simulink model "code_group46"  (R2022b)
settings: Solver=FixedStepAuto  StartTime=0.0  StopTime=2  FixedStep=1e-3  RelTol=1e-3  EnableMultiTasking=on
undefined symbols (not defined in the file): A0, A1, D0, D1, D10, D11, D12, D13, D2, D3, D4, D5, D6, D7, D8, D9, PTA0, PTA1, PTA2, PTB2, PTB23, PTB3, PTB9, PTC16, PTC17, PTC2, PTC3, PTC4, PTD0, PTD1, PTD2, PTD3
libraries: frdmk64flib x19, etargetslib x19, simulink x2
(part 1 of 2)
settings Model: ExtModeTrigDuration=5  Creator=aliciamorielli  LastModifiedBy=kavya
settings SolverCC: AlgebraicLoopSolver=TrustRegion
settings OptimizationCC: EnhancedBackFolding=on  PassReuseOutputArgsThreshold=0  MaxStackSize=64  OptimizeBlockOrder=speed  DifferentSizesBufferReuse=on  OptimizationCustomize=off
settings DebuggingCC: ParameterTunabilityLossMsg=error  UnconnectedInputMsg=warning  UnconnectedOutputMsg=warning  UnconnectedLineMsg=warning  SFMachineParentedDataDiag=warning
settings HardwareCC: ProdBitPerPointer=32  ProdBitPerSizeT=32  ProdBitPerPtrDiffT=32  ProdLargestAtomicInteger=Long  ProdLargestAtomicFloat=Double  ProdWordSize=32  ProdHWDeviceType=ARM Compatible->ARM Cortex  UseEmbeddedCoderFeatures=off
settings ModelReferenceCC: EnableRefExpFcnMdlSchedulingChecks=on
settings SFSimCC: MATLABDynamicMemAlloc=off
settings RTWCC: Description=Embedded Coder  SystemTargetFile=ert.tlc  HardwareBoard=NXP FRDM-K64F  TLCOptions="-aInlineSetEventsForThisBaseRateFcn=TLC_FALSE -aSuppressMultiTaskScheduler=TLC_FALSE  -aRateBasedStepFcn=0"  TemplateMakefile=ert_default_tmf  Toolchain=GNU Tools for ARM Embedded Processors  DLArmComputeVersion=19.05
settings CodeAppCC: ForceParamTrailComments=on  OperatorAnnotations=on
settings ERTTargetCC: ERTCustomFileBanners=off  SupportContinuousTime=on  SupportNonInlinedSFcns=on  RemoveResetFunc=off  ModelStepFunctionPrototypeControlCompliant=off  ExtModeTransport=4  ExtModeMexFile=sendToCommService

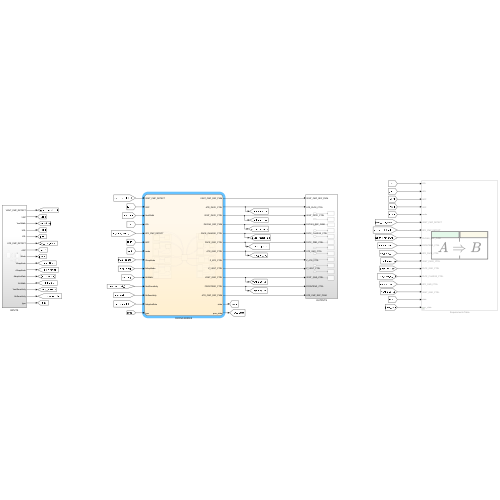
[thumbnail: Simulink's stored preview of the top-level diagram]
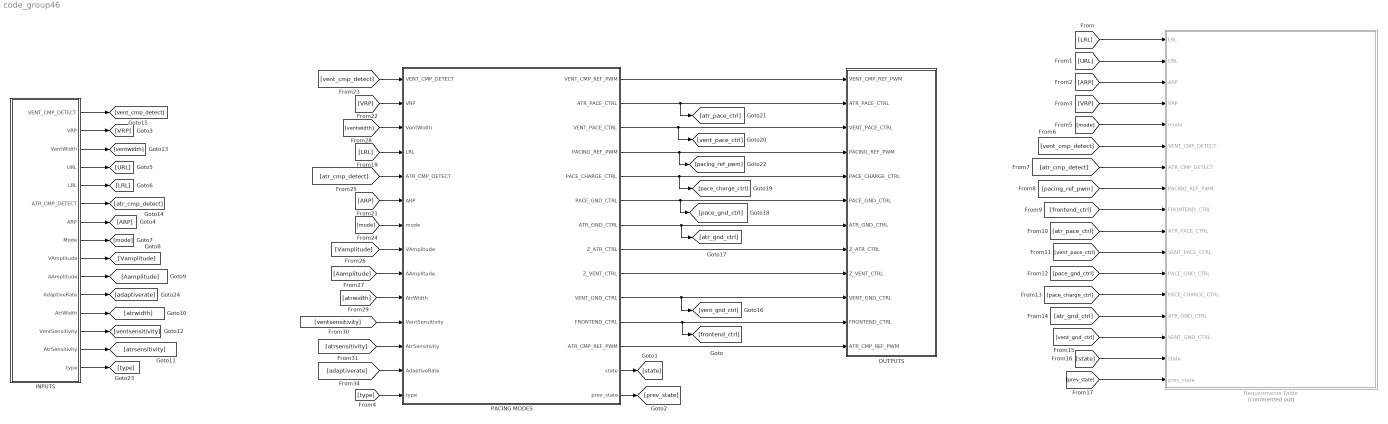
== system code_group46 ==
  INPUTS : Subsystem
  OUTPUTS : Subsystem
  PACING MODES : Stateflow chart  TreatAsAtomicUnit=on
      settings: PortSchema="{\"entries\":[{\"content\":{\"sides\":[{\"content\":{\"connectorIds\":[\"In1\",\"In4\",\"In2\",\"In3\",\"In6\",\"In5\",\"In7\",\"In8\",\"In9\",\"In10\",\"In11\",\"In12\",\"In13\",\"In14\"]},\"type\":\"ConnectorPlacement.EquallySpacedRectSide\",\"uuid\":\"24afec03-bc13-4065-9064-27bef3c43f7a\"},{\"content\":{\"connectorIds\":[\"Out11\",\"Out1\",\"Out2\",\"Out3\",\"Out4\",\"Out5\",\"Out6\",\"Out7\",\"Out8\",\"Out9\",\"Out10\",\"Out12\",\"Out13\",\"Out14\"],\"side\":\"RIGHT\"},\"type\":\"ConnectorPlacement.EquallySpacedRectSide\",\"uuid\":\"79d0ee85-df22-4c09-8ba8-cd763efde854\"},{\"content\":{\"connectorIds\":[],\"side\":\"TOP\"},\"type\":\"ConnectorPlacement.EquallySpacedRectSide\",\"uuid\":\"d342e713-b0ae-4b06-a4c2-9648f7d82d61\"},{\"content\":{\"connectorIds\":[],\"side\":\"BOTTOM\"},\"type\":\"ConnectorPlacement.EquallySpacedRectSide\",\"uuid\":\"4b63818c-7bd6-427f-a568-d3913931a17b\"}]},\"type\":\"ConnectorPlacement.EquallySpacedConnector\",\"uuid\":\"408ec0d3-1c59-4342-b3c9-42fd185f3962\"}],\"packageUris\":[\"http://schema.mathworks.com/mf0/Connector/R2020b\"],\"version\":\"1.0\"}"
  Requirements Table : Requirements Table  Commented=on  TreatAsAtomicUnit=on
  wires:
  PACING MODES/11(VENT_CMP_REF_PWM) -> OUTPUTS/1(VENT_CMP_REF_PWM)
  PACING MODES/2(VENT_PACE_CTRL) -> [vent_pace_ctrl], OUTPUTS/3(VENT_PACE_CTRL)
  PACING MODES/3(PACING_REF_PWM) -> [pacing_ref_pwm], OUTPUTS/4(PACING_REF_PWM)
  PACING MODES/4(PACE_CHARGE_CTRL) -> [pace_charge_ctrl], OUTPUTS/5(PACE_CHARGE_CTRL)
  PACING MODES/5(PACE_GND_CTRL) -> [pace_gnd_ctrl], OUTPUTS/6(PACE_GND_CTRL)
  PACING MODES/6(ATR_GND_CTRL) -> [atr_gnd_ctrl], OUTPUTS/7(ATR_GND_CTRL)
  PACING MODES/7(Z_ATR_CTRL) -> OUTPUTS/8(Z_ATR_CTRL)
  PACING MODES/8(Z_VENT_CTRL) -> OUTPUTS/9(Z_VENT_CTRL)
  PACING MODES/9(VENT_GND_CTRL) -> [vent_gnd_ctrl], OUTPUTS/10(VENT_GND_CTRL)
  PACING MODES/10(FRONTEND_CTRL) -> [frontend_ctrl], OUTPUTS/11(FRONTEND_CTRL)
  PACING MODES/12(ATR_CMP_REF_PWM) -> OUTPUTS/12(ATR_CMP_REF_PWM)
  PACING MODES/1(ATR_PACE_CTRL) -> [atr_pace_ctrl], OUTPUTS/2(ATR_PACE_CTRL)
  [LRL] -> Requirements Table/1(LRL)
  [URL] -> Requirements Table/2(URL)
  [ARP] -> Requirements Table/3(ARP)
  [VRP] -> Requirements Table/4(VRP)
  [mode] -> Requirements Table/5(mode)
  [vent_cmp_detect] -> Requirements Table/6(VENT_CMP_DETECT)
  [atr_cmp_detect] -> Requirements Table/7(ATR_CMP_DETECT)
  [pacing_ref_pwm] -> Requirements Table/8(PACING_REF_PWM)
  [frontend_ctrl] -> Requirements Table/9(FRONTEND_CTRL)
  [atr_pace_ctrl] -> Requirements Table/10(ATR_PACE_CTRL)
  [vent_pace_ctrl] -> Requirements Table/11(VENT_PACE_CTRL)
  [pace_gnd_ctrl] -> Requirements Table/12(PACE_GND_CTRL)
  [pace_charge_ctrl] -> Requirements Table/13(PACE_CHARGE_CTRL)
  [atr_gnd_ctrl] -> Requirements Table/14(ATR_GND_CTRL)
  [vent_gnd_ctrl] -> Requirements Table/15(VENT_GND_CTRL)
  [state] -> Requirements Table/16(state)
  [prev_state] -> Requirements Table/17(prev_state)
  PACING MODES/13(state) -> [state]
  PACING MODES/14(prev_state) -> [prev_state]
  [LRL] -> PACING MODES/3(LRL)
  [ARP] -> PACING MODES/5(ARP)
  [VRP] -> PACING MODES/4(VRP)
  [mode] -> PACING MODES/7(mode)
  [vent_cmp_detect] -> PACING MODES/1(VENT_CMP_DETECT)
  [atr_cmp_detect] -> PACING MODES/6(ATR_CMP_DETECT)
  [Vamplitude] -> PACING MODES/8(VAmplitude)
  [Aamplitude] -> PACING MODES/9(AAmplitude)
  INPUTS/2(VRP) -> [VRP]
  INPUTS/7(ARP) -> [ARP]
  INPUTS/3(VentWidth) -> [ventwidth]
  INPUTS/5(LRL) -> [LRL]
  INPUTS/8(Mode) -> [mode]
  INPUTS/9(VAmplitude) -> [Vamplitude]
  INPUTS/10(AAmplitude) -> [Aamplitude]
  INPUTS/13(VentSensitivity) -> [ventsensitivity]
  INPUTS/14(AtrSensitivity) -> [atrsensitivity]
  INPUTS/12(AtrWidth) -> [atrwidth]
  [ventwidth] -> PACING MODES/2(VentWidth)
  [atrwidth] -> PACING MODES/10(AtrWidth)
  INPUTS/1(VENT_CMP_DETECT) -> [vent_cmp_detect]
  INPUTS/6(ATR_CMP_DETECT) -> [atr_cmp_detect]
  [ventsensitivity] -> PACING MODES/11(VentSensitivity)
  [atrsensitivity] -> PACING MODES/12(AtrSensitivity)
  INPUTS/4(URL) -> [URL]
  INPUTS/11(AdaptiveRate) -> [adaptiverate]
  [adaptiverate] -> PACING MODES/13(AdaptiveRate)
  [type] -> PACING MODES/14(type)
  INPUTS/15(type) -> [type]

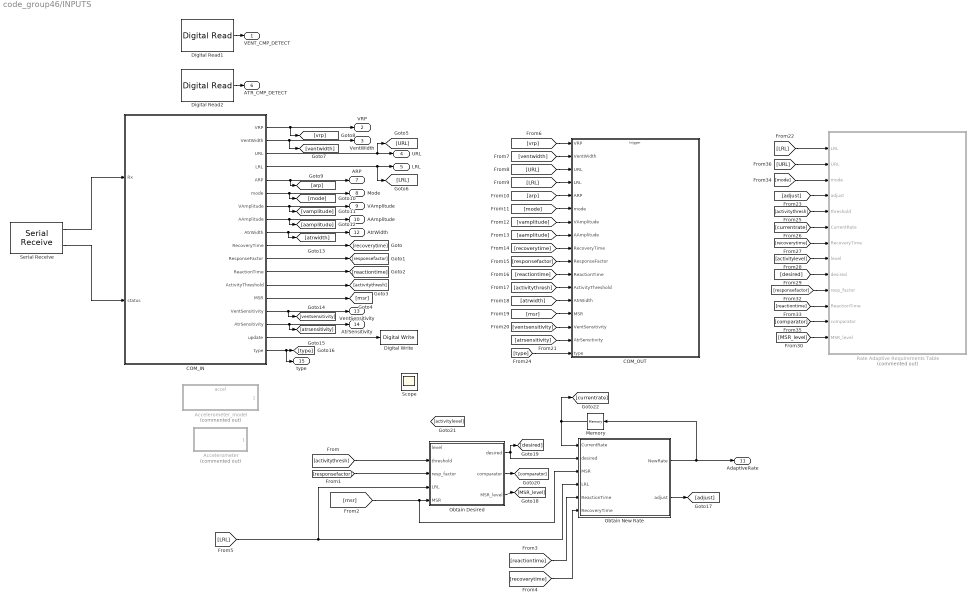
== system code_group46/INPUTS ==
  Accelerometer : Subsystem  Commented=on  ReferencedSubsystem=accelerometer
  Accelerometer_model : ModelReference  Commented=on  ModelNameDialog=accel  SimulationMode=Normal  ModelReferenceVersion=2.0
  COM_IN : Stateflow chart  TreatAsAtomicUnit=on
      settings: PortSchema="{\"entries\":[{\"content\":{\"sides\":[{\"content\":{\"connectorIds\":[\"In1\",\"In2\"]},\"type\":\"ConnectorPlacement.EquallySpacedRectSide\",\"uuid\":\"eafe7878-2647-49a4-97cb-41e68478fa40\"},{\"content\":{\"connectorIds\":[\"Out3\",\"Out1\",\"Out5\",\"Out6\",\"Out7\",\"Out2\",\"Out4\",\"Out8\",\"Out13\",\"Out9\",\"Out10\",\"Out11\",\"Out12\",\"Out14\",\"Out15\",\"Out16\",\"Out17\",\"Out18\"],\"side\":\"RIGHT\"},\"type\":\"ConnectorPlacement.EquallySpacedRectSide\",\"uuid\":\"c0ba33de-ccdc-4037-9e5a-c304987946dd\"},{\"content\":{\"connectorIds\":[],\"side\":\"TOP\"},\"type\":\"ConnectorPlacement.EquallySpacedRectSide\",\"uuid\":\"204d3e33-d140-4353-8067-53c664c1cb64\"}]},\"type\":\"ConnectorPlacement.EquallySpacedConnector\",\"uuid\":\"8b254745-690b-4cb1-aa57-728c67132f0f\"}],\"packageUris\":[\"http://schema.mathworks.com/mf0/Connector/R2020b\"],\"version\":\"1.0\"}"
  COM_OUT : Subsystem  TreatAsAtomicUnit=on
  Digital Read1 : frdmk64flib/Digital Read  Whichpin=PTC17 (D1)  SampleTime=-1
  Digital Read2 : frdmk64flib/Digital Read  Whichpin=PTC16 (D0)  SampleTime=-1
  Digital Write : frdmk64flib/Digital Write  Whichpin=RED_LED
  Memory : Memory  InheritSampleTime=on
  Obtain Desired : Stateflow chart  TreatAsAtomicUnit=on
      settings: PortSchema="{\"entries\":[{\"content\":{\"sides\":[{\"content\":{\"connectorIds\":[\"In3\",\"In1\",\"In2\",\"In5\",\"In4\"]},\"type\":\"ConnectorPlacement.EquallySpacedRectSide\",\"uuid\":\"5c134849-3d1d-4c56-8571-ceae08da9f45\"},{\"content\":{\"connectorIds\":[\"Out1\",\"Out2\",\"Out3\"],\"side\":\"RIGHT\"},\"type\":\"ConnectorPlacement.EquallySpacedRectSide\",\"uuid\":\"7618640d-b82a-4535-8229-36335d1597eb\"},{\"content\":{\"connectorIds\":[],\"side\":\"TOP\"},\"type\":\"ConnectorPlacement.EquallySpacedRectSide\",\"uuid\":\"2f785ce6-cbe7-41ad-b744-28eba0ea0bcd\"}]},\"type\":\"ConnectorPlacement.EquallySpacedConnector\",\"uuid\":\"c0de53b0-65a0-4d09-8942-b2384056cc94\"}],\"packageUris\":[\"http://schema.mathworks.com/mf0/Connector/R2020b\"],\"version\":\"1.0\"}"
  Obtain New Rate : Stateflow chart  TreatAsAtomicUnit=on
      settings: PortSchema="{\"entries\":[{\"content\":{\"sides\":[{\"content\":{\"connectorIds\":[\"In2\",\"In1\",\"In5\",\"In6\",\"In3\",\"In4\"]},\"type\":\"ConnectorPlacement.EquallySpacedRectSide\",\"uuid\":\"1d91cfe0-cd55-4bdf-aa16-d6a917e51e7e\"},{\"content\":{\"connectorIds\":[\"Out1\",\"Out2\"],\"side\":\"RIGHT\"},\"type\":\"ConnectorPlacement.EquallySpacedRectSide\",\"uuid\":\"e994e035-8773-49d5-b660-bbaeb9e2bece\"},{\"content\":{\"connectorIds\":[],\"side\":\"TOP\"},\"type\":\"ConnectorPlacement.EquallySpacedRectSide\",\"uuid\":\"300aa799-ec86-4945-b5cc-5c980ffddaca\"}]},\"type\":\"ConnectorPlacement.EquallySpacedConnector\",\"uuid\":\"358a8051-88ab-49cd-8e65-a99c6960b963\"}],\"packageUris\":[\"http://schema.mathworks.com/mf0/Connector/R2020b\"],\"version\":\"1.0\"}"
  Rate Adaptive Requirements Table : Requirements Table  Commented=on  TreatAsAtomicUnit=on
  Scope : Scope
  Serial Receive : frdmk64flib/Serial Receive  SCIModule=0  Baudrate=uint32(9600)  Parity=None  StopBits=1  HardwareFlowControl=None  ByteOrder=LittleEndian  DataType=uint8  DataLength=112  BlockingMode=off  OutputStatus=on  SampleTime=-1
  VENT_CMP_DETECT : Outport  OutDataTypeStr=boolean
  VRP : Outport  Port=2  OutDataTypeStr=double
  VentWidth : Outport  Port=3  OutDataTypeStr=int16
  URL : Outport  Port=4  OutDataTypeStr=double
  LRL : Outport  Port=5  OutDataTypeStr=double
  ATR_CMP_DETECT : Outport  Port=6  OutDataTypeStr=boolean
  ARP : Outport  Port=7  OutDataTypeStr=double
  Mode : Outport  Port=8  OutDataTypeStr=int16
  VAmplitude : Outport  Port=9  OutDataTypeStr=double
  AAmplitude : Outport  Port=10  OutDataTypeStr=double
  AdaptiveRate : Outport  Port=11
  AtrWidth : Outport  Port=12  OutDataTypeStr=int16
  VentSensitivity : Outport  Port=13
  AtrSensitivity : Outport  Port=14
  type : Outport  Port=15
  wires:
  COM_IN/5(URL) -> URL/1, [URL]
  COM_IN/1(VentWidth) -> [ventwidth], VentWidth/1
  Digital Read1/1 -> VENT_CMP_DETECT/1
  COM_IN/3(VRP) -> [vrp], VRP/1
  COM_IN/7(ARP) -> [arp], ARP/1
  Digital Read2/1 -> ATR_CMP_DETECT/1
  COM_IN/2(mode) -> [mode], Mode/1
  COM_IN/4(VAmplitude) -> [vamplitude], VAmplitude/1
  COM_IN/8(AAmplitude) -> [aamplitude], AAmplitude/1
  [activitythresh] -> Obtain Desired/1(threshold)
  [msr] -> Obtain New Rate/5(MSR), Obtain Desired/4(MSR)
  [LRL] -> Obtain New Rate/6(LRL), Obtain Desired/5(LRL)
  COM_IN/6(LRL) -> [LRL], LRL/1
  Obtain Desired/1(desired) -> Obtain New Rate/1(desired), [desired]
  [reactiontime] -> Obtain New Rate/3(ReactionTime)
  [recoverytime] -> Obtain New Rate/4(RecoveryTime)
  Obtain New Rate/1(NewRate) -> Memory/1, AdaptiveRate/1
  Obtain New Rate/2(adjust) -> [adjust]
  Serial Receive/2 -> COM_IN/2(status)
  Serial Receive/1 -> COM_IN/1(Rx)
  COM_IN/13(AtrWidth) -> [atrwidth], AtrWidth/1
  COM_IN/9(RecoveryTime) -> [recoverytime]
  COM_IN/10(ResponseFactor) -> [responsefactor]
  COM_IN/11(ReactionTime) -> [reactiontime]
  COM_IN/12(ActivityThreshold) -> [activitythresh]
  COM_IN/14(MSR) -> [msr]
  COM_IN/16(AtrSensitivity) -> [atrsensitivity], AtrSensitivity/1
  COM_IN/15(VentSensitivity) -> [ventsensitivity], VentSensitivity/1
  [ventwidth] -> COM_OUT/2(VentWidth)
  [vrp] -> COM_OUT/1(VRP)
  [URL] -> COM_OUT/3(URL)
  [LRL] -> COM_OUT/4(LRL)
  [arp] -> COM_OUT/5(ARP)
  [mode] -> COM_OUT/6(mode)
  [vamplitude] -> COM_OUT/7(VAmplitude)
  [aamplitude] -> COM_OUT/8(AAmplitude)
  [recoverytime] -> COM_OUT/9(RecoveryTime)
  [responsefactor] -> COM_OUT/10(ResponseFactor)
  [reactiontime] -> COM_OUT/11(ReactionTime)
  [activitythresh] -> COM_OUT/12(ActivityThreshold)
  [atrwidth] -> COM_OUT/13(AtrWidth)
  [msr] -> COM_OUT/14(MSR)
  [ventsensitivity] -> COM_OUT/15(VentSensitivity)
  [atrsensitivity] -> COM_OUT/16(AtrSensitivity)
  Memory/1 -> [currentrate], Obtain New Rate/2(CurrentRate)
  [LRL] -> Rate Adaptive Requirements Table/1(LRL)
  [mode] -> Rate Adaptive Requirements Table/3(mode)
  [responsefactor] -> Obtain Desired/2(resp_factor)
  Obtain Desired/2(comparator) -> [comparator]
  [adjust] -> Rate Adaptive Requirements Table/4(adjust)
  [activitythresh] -> Rate Adaptive Requirements Table/5(threshold)
  [currentrate] -> Rate Adaptive Requirements Table/6(CurrentRate)
  [recoverytime] -> Rate Adaptive Requirements Table/7(RecoveryTime)
  [activitylevel] -> Rate Adaptive Requirements Table/8(level)
  [desired] -> Rate Adaptive Requirements Table/9(desired)
  [responsefactor] -> Rate Adaptive Requirements Table/10(resp_factor)
  [reactiontime] -> Rate Adaptive Requirements Table/11(ReactionTime)
  [comparator] -> Rate Adaptive Requirements Table/12(comparator)
  [URL] -> Rate Adaptive Requirements Table/2(URL)
  COM_IN/17(update) -> Digital Write/1
  COM_IN/18(type) -> type/1, [type]
  [type] -> COM_OUT/17(type)
  Obtain Desired/3(MSR_level) -> [MSR_level]
  [MSR_level] -> Rate Adaptive Requirements Table/13(MSR_level)

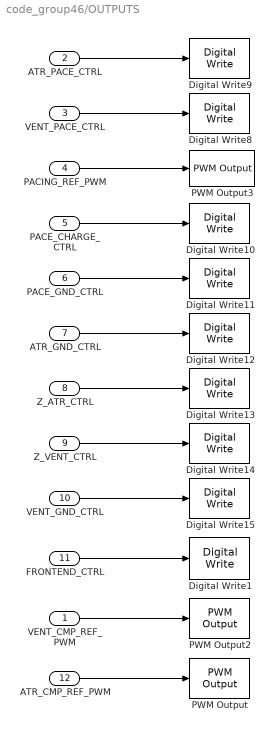
== system code_group46/OUTPUTS ==
  VENT_CMP_REF_PWM : Inport  OutDataTypeStr=double
  ATR_PACE_CTRL : Inport  Port=2  OutDataTypeStr=boolean
  VENT_PACE_CTRL : Inport  Port=3  OutDataTypeStr=boolean
  PACING_REF_PWM : Inport  Port=4  OutDataTypeStr=double
  PACE_CHARGE_CTRL : Inport  Port=5  OutDataTypeStr=boolean
  PACE_GND_CTRL : Inport  Port=6  OutDataTypeStr=boolean
  ATR_GND_CTRL : Inport  Port=7  OutDataTypeStr=boolean
  Z_ATR_CTRL : Inport  Port=8  OutDataTypeStr=boolean
  Z_VENT_CTRL : Inport  Port=9  OutDataTypeStr=boolean
  VENT_GND_CTRL : Inport  Port=10  OutDataTypeStr=boolean
  FRONTEND_CTRL : Inport  Port=11  OutDataTypeStr=boolean
  ATR_CMP_REF_PWM : Inport  Port=12  OutDataTypeStr=double
  Digital Write1 : frdmk64flib/Digital Write  Whichpin=PTD1 (D13)
  Digital Write10 : frdmk64flib/Digital Write  Whichpin=PTB9 (D2)
  Digital Write11 : frdmk64flib/Digital Write  Whichpin=PTD0 (D10)
  Digital Write12 : frdmk64flib/Digital Write  Whichpin=PTD2 (D11)
  Digital Write13 : frdmk64flib/Digital Write  Whichpin=PTB23 (D4)
  Digital Write14 : frdmk64flib/Digital Write  Whichpin=PTC3 (D7)
  Digital Write15 : frdmk64flib/Digital Write  Whichpin=PTD3 (D12)
  Digital Write8 : frdmk64flib/Digital Write  Whichpin=PTC4 (D9)
  Digital Write9 : frdmk64flib/Digital Write  Whichpin=PTA0 (D8)
  PWM Output : frdmk64flib/PWM Output  Whichpin=PTC2 (D6)  InitialFrequency=2000  InitialDutyCycle=53
  PWM Output2 : frdmk64flib/PWM Output  Whichpin=PTA1 (D3)  InitialFrequency=2000  InitialDutyCycle=70
  PWM Output3 : frdmk64flib/PWM Output  Whichpin=PTA2 (D5)  InitialFrequency=2000  InitialDutyCycle=40
  wires:
  Z_ATR_CTRL/1 -> Digital Write13/1
  Z_VENT_CTRL/1 -> Digital Write14/1
  FRONTEND_CTRL/1 -> Digital Write1/1
  PACE_CHARGE_CTRL/1 -> Digital Write10/1
  VENT_PACE_CTRL/1 -> Digital Write8/1
  ATR_CMP_REF_PWM/1 -> PWM Output/1
  VENT_CMP_REF_PWM/1 -> PWM Output2/1
  ATR_GND_CTRL/1 -> Digital Write12/1
  ATR_PACE_CTRL/1 -> Digital Write9/1
  VENT_GND_CTRL/1 -> Digital Write15/1
  PACE_GND_CTRL/1 -> Digital Write11/1
  PACING_REF_PWM/1 -> PWM Output3/1

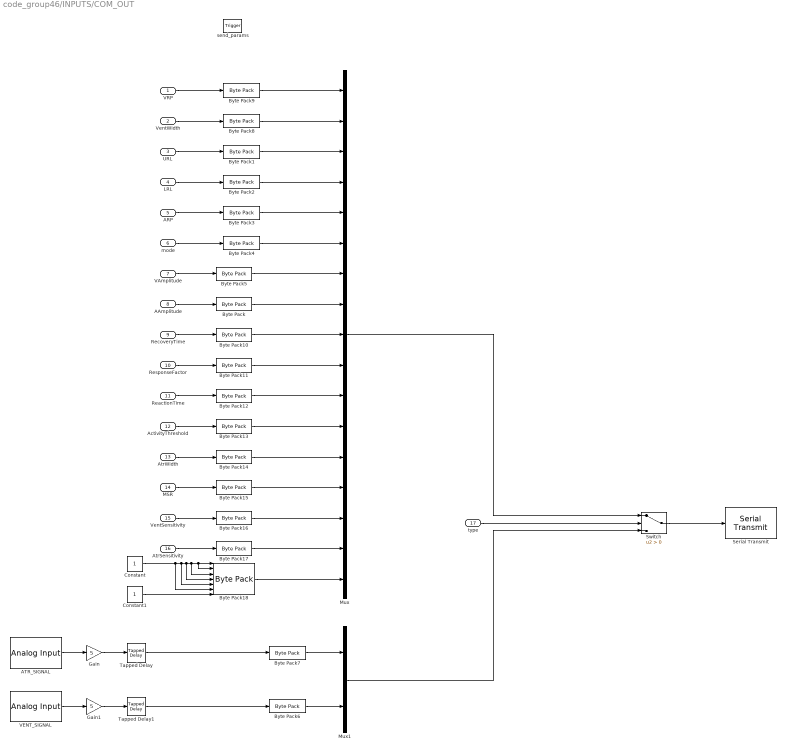
== system code_group46/INPUTS/COM_OUT ==
  VRP : Inport  OutDataTypeStr=double
  VentWidth : Inport  Port=2  OutDataTypeStr=int16
  URL : Inport  Port=3  OutDataTypeStr=double
  LRL : Inport  Port=4  OutDataTypeStr=double
  ARP : Inport  Port=5  OutDataTypeStr=double
  mode : Inport  Port=6  OutDataTypeStr=int16
  VAmplitude : Inport  Port=7  OutDataTypeStr=double
  AAmplitude : Inport  Port=8  OutDataTypeStr=double
  RecoveryTime : Inport  Port=9  OutDataTypeStr=double
  ResponseFactor : Inport  Port=10  OutDataTypeStr=double
  ReactionTime : Inport  Port=11  OutDataTypeStr=double
  ActivityThreshold : Inport  Port=12  OutDataTypeStr=double
  AtrWidth : Inport  Port=13  OutDataTypeStr=int16
  MSR : Inport  Port=14  OutDataTypeStr=double
  VentSensitivity : Inport  Port=15  OutDataTypeStr=double
  AtrSensitivity : Inport  Port=16  OutDataTypeStr=double
  type : Inport  Port=17
  send_params : TriggerPort  TriggerType=function-call  IsSimulinkFunction=on  FunctionName=send_params  VariantControl=(inherit)
  ATR_SIGNAL : frdmk64flib/Analog Input  Whichpin=PTB2 (A0)  SampleTime=-1
  Byte Pack{,1..3,5..7,9..13,15..17} (15 alike) : etargetslib/Byte Pack  datatypes={'double'}  byteAlign=1
  Byte Pack14 : etargetslib/Byte Pack  datatypes={'int16'}  byteAlign=1
  Byte Pack18 : etargetslib/Byte Pack  datatypes={'double','double','double','double','double','double','int16'}  byteAlign=1
  Byte Pack4 : etargetslib/Byte Pack  datatypes={'int16'}  byteAlign=1
  Byte Pack8 : etargetslib/Byte Pack  datatypes={'int16'}  byteAlign=1
  Constant : Constant  OutDataTypeStr=double
  Constant1 : Constant  OutDataTypeStr=int16
  Gain : Gain  Gain=5
  Gain1 : Gain  Gain=5
  Mux : Mux  Inputs=17
  Mux1 : Mux  Inputs=2
  Serial Transmit : frdmk64flib/Serial Transmit  SCIModule=0  Baudrate=uint32(9600)  Parity=None  StopBits=1  HardwareFlowControl=None  ByteOrder=LittleEndian  BlockingMode=on  OutputStatus=off
  Switch : Switch  Criteria=u2 > Threshold  SaturateOnIntegerOverflow=off  InputSameDT=off
  Tapped Delay : simulink/Discrete/Tapped Delay  vinit=0.0  samptime=-1  NumDelays=10  DelayOrder=Oldest  includeCurrent=off
  Tapped Delay1 : simulink/Discrete/Tapped Delay  vinit=0.0  samptime=-1  NumDelays=10  DelayOrder=Oldest  includeCurrent=off
  VENT_SIGNAL : frdmk64flib/Analog Input  Whichpin=PTB3 (A1)  SampleTime=-1
  wires:
  AAmplitude/1 -> Byte Pack/1
  VAmplitude/1 -> Byte Pack5/1
  mode/1 -> Byte Pack4/1
  ARP/1 -> Byte Pack3/1
  LRL/1 -> Byte Pack2/1
  URL/1 -> Byte Pack1/1
  VentWidth/1 -> Byte Pack8/1
  VRP/1 -> Byte Pack9/1
  Byte Pack/1 -> Mux/8
  Byte Pack5/1 -> Mux/7
  Byte Pack4/1 -> Mux/6
  Byte Pack3/1 -> Mux/5
  Byte Pack2/1 -> Mux/4
  Byte Pack1/1 -> Mux/3
  Byte Pack8/1 -> Mux/2
  Byte Pack9/1 -> Mux/1
  RecoveryTime/1 -> Byte Pack10/1
  ResponseFactor/1 -> Byte Pack11/1
  ReactionTime/1 -> Byte Pack12/1
  ActivityThreshold/1 -> Byte Pack13/1
  AtrWidth/1 -> Byte Pack14/1
  MSR/1 -> Byte Pack15/1
  Byte Pack10/1 -> Mux/9
  Byte Pack11/1 -> Mux/10
  Byte Pack12/1 -> Mux/11
  Byte Pack13/1 -> Mux/12
  Byte Pack14/1 -> Mux/13
  Byte Pack15/1 -> Mux/14
  VentSensitivity/1 -> Byte Pack16/1
  AtrSensitivity/1 -> Byte Pack17/1
  Byte Pack17/1 -> Mux/16
  Byte Pack16/1 -> Mux/15
  Mux/1 -> Switch/1
  Switch/1 -> Serial Transmit/1
  ATR_SIGNAL/1 -> Gain/1
  VENT_SIGNAL/1 -> Gain1/1
  Byte Pack7/1 -> Mux1/1
  Byte Pack6/1 -> Mux1/2
  Mux1/1 -> Switch/3
  type/1 -> Switch/2
  Gain/1 -> Tapped Delay/1
  Gain1/1 -> Tapped Delay1/1
  Tapped Delay/1 -> Byte Pack7/1
  Tapped Delay1/1 -> Byte Pack6/1
  Constant/1 -> Byte Pack18/6, Byte Pack18/5, Byte Pack18/4, Byte Pack18/3, Byte Pack18/2, Byte Pack18/1
  Byte Pack18/1 -> Mux/17
  Constant1/1 -> Byte Pack18/7

== stateflow chart code_group46/INPUTS/Rate Adaptive Requirements Table ==
  (default) -> (junction 1073758337)
  (junction 1073758337) -> (junction 1073758338) : {
      | % SF_REQ_REV_07
      | }
  (junction 1073758338) -> (junction 1073758340) : {
      | % HEADER_ASSIGNMENTS
      |
      | }
  (junction 1073758340) -> (junction 1073758342) : {
      | % START_A_4
      | }
  (junction 1073758342) -> (junction 1073758344) : {
      | }
  (junction 1073758344) -> (junction 1073758346) : {
      | reqtable_assumption((LRL <= 175 && LRL >= 30 && LRL <= URL), 4);
      | }
  (junction 1073758346) -> (junction 1073758348) : {
      | }
  (junction 1073758348) -> (junction 1073758350) : {
      | % END_A_4
      | }
  (junction 1073758350) -> (junction 1073758352) : {
      | % START_A_7
      | }
  (junction 1073758352) -> (junction 1073758354) : {
      | }
  (junction 1073758354) -> (junction 1073758356) : {
      | reqtable_assumption((URL <= 175 && URL >= 50), 7);
      | }
  (junction 1073758356) -> (junction 1073758358) : {
      | }
  (junction 1073758358) -> (junction 1073758360) : {
      | % END_A_7
      | }
  (junction 1073758360) -> (junction 1073758362) : {
      | % START_A_10
      | }
  (junction 1073758362) -> (junction 1073758364) : {
      | }
  (junction 1073758364) -> (junction 1073758366) : {
      | reqtable_assumption((RecoveryTime >=120 && RecoveryTime <= 960), 10);
      | }
  (junction 1073758366) -> (junction 1073758368) : {
      | }
  (junction 1073758368) -> (junction 1073758370) : {
      | % END_A_10
      | }
  (junction 1073758370) -> (junction 1073758372) : {
      | % START_A_16
      | }
  (junction 1073758372) -> (junction 1073758374) : {
      | }
  (junction 1073758374) -> (junction 1073758376) : {
      | reqtable_assumption((resp_factor>=1 && resp_factor<=16), 16);
      | }
  (junction 1073758376) -> (junction 1073758378) : {
      | }
  (junction 1073758378) -> (junction 1073758380) : {
      | % END_A_16
      | }
  (junction 1073758380) -> (junction 1073758382) : {
      | % START_A_19
      | }
  (junction 1073758382) -> (junction 1073758384) : {
      | }
  (junction 1073758384) -> (junction 1073758386) : {
      | reqtable_assumption((ReactionTime >=10 && ReactionTime<=50), 19);
      | }
  (junction 1073758386) -> (junction 1073758388) : {
      | }
  (junction 1073758388) -> (junction 1073758390) : {
      | % END_A_19
      | }
  (junction 1073758390) -> (junction 1073758392) : {
      | % START_A_22
      | }
  (junction 1073758392) -> (junction 1073758394) : {
      | }
  (junction 1073758394) -> (junction 1073758396) : {
      | reqtable_assumption((mode >= 0 && mode <= 8), 22);
      | }
  (junction 1073758396) -> (junction 1073758398) : {
      | }
  (junction 1073758398) -> (junction 1073758400) : {
      | % END_A_22
      | }
  (junction 1073758400) -> (junction 1073758402) : {
      | % START_R_133
      | }
  (junction 1073758402) -> (junction 1073758404) : {
      | }
  (junction 1073758404) -> (junction 1073758406)
  (junction 1073758406) -> (junction 1073758408) [order 1] : [(((mode) == (5)) || ((mode) == (6)) || ((mode) == (7)) || ((mode) == (8)))]
  (junction 1073758406) -> (junction 1073758468) [order 2]
  (junction 1073758408) -> (junction 1073758410) : {
      |
      |
      | }
  (junction 1073758410) -> (junction 1073758412) : {
      | }
  (junction 1073758412) -> (junction 1073758414) : {
      | % START_R_136
      | }
  (junction 1073758414) -> (junction 1073758416) : {
      | }
  (junction 1073758416) -> (junction 1073758418)
  (junction 1073758418) -> (junction 1073758420) [order 1] : [(((level<=threshold) == (true))) && (((level>threshold && level < MSR_level) == (false))) && (((level>=MSR_level) == (false)))]
  (junction 1073758418) -> (junction 1073758426) [order 2]
  (junction 1073758420) -> (junction 1073758422) : {
      | reqtable_postcondition((((comparator) == ("below"))), 'R:1.1');
      |
      |
      | }
  (junction 1073758422) -> (junction 1073758424) : {
      | }
  (junction 1073758424) -> (junction 1073758426)
  (junction 1073758426) -> (junction 1073758428)
  (junction 1073758428) -> (junction 1073758430) : {
      | % END_R_136
      | }
  (junction 1073758430) -> (junction 1073758432) : {
      | % START_R_139
      | }
  (junction 1073758432) -> (junction 1073758434) : {
      | }
  (junction 1073758434) -> (junction 1073758436)
  (junction 1073758436) -> (junction 1073758438) [order 1] : [(((level<=threshold) == (false))) && (((level>threshold && level < MSR_level) == (true))) && (((level>=MSR_level) == (false)))]
  (junction 1073758436) -> (junction 1073758444) [order 2]
  (junction 1073758438) -> (junction 1073758440) : {
      | reqtable_postcondition((((comparator) == ("within"))), 'R:1.2');
      |
      |
      | }
  (junction 1073758440) -> (junction 1073758442) : {
      | }
  (junction 1073758442) -> (junction 1073758444)
  (junction 1073758444) -> (junction 1073758446)
  (junction 1073758446) -> (junction 1073758448) : {
      | % END_R_139
      | }
  (junction 1073758448) -> (junction 1073758450) : {
      | % START_R_142
      | }
  (junction 1073758450) -> (junction 1073758452) : {
      | }
  (junction 1073758452) -> (junction 1073758454)
  (junction 1073758454) -> (junction 1073758456) [order 1] : [(((level<=threshold) == (false))) && (((level>threshold && level < MSR_level) == (false))) && (((level>=MSR_level) == (true)))]
  (junction 1073758454) -> (junction 1073758462) [order 2]
  (junction 1073758456) -> (junction 1073758458) : {
      | reqtable_postcondition((((comparator) == ("above"))), 'R:1.3');
      |
      |
      | }
  (junction 1073758458) -> (junction 1073758460) : {
      | }
  (junction 1073758460) -> (junction 1073758462)
  (junction 1073758462) -> (junction 1073758464)
  (junction 1073758464) -> (junction 1073758466) : {
      | % END_R_142
      | }
  (junction 1073758466) -> (junction 1073758468)
  (junction 1073758468) -> (junction 1073758470)
  (junction 1073758470) -> (junction 1073758472) : {
      | % END_R_133
      | }
  (junction 1073758472) -> (junction 1073758474) : {
      | % START_R_145
      | }
  (junction 1073758474) -> (junction 1073758476) : {
      | }
  (junction 1073758476) -> (junction 1073758478)
  (junction 1073758478) -> (junction 1073758480) [order 1] : [(((mode) == (5)) || ((mode) == (6)) || ((mode) == (7)) || ((mode) == (8)))]
  (junction 1073758478) -> (junction 1073758540) [order 2]
  (junction 1073758480) -> (junction 1073758482) : {
      |
      |
      | }
  (junction 1073758482) -> (junction 1073758484) : {
      | }
  (junction 1073758484) -> (junction 1073758486) : {
      | % START_R_148
      | }
  (junction 1073758486) -> (junction 1073758488) : {
      | }
  (junction 1073758488) -> (junction 1073758490)
  (junction 1073758490) -> (junction 1073758492) [order 1] : [(((desired<CurrentRate) == (true))) && (((desired>CurrentRate) == (false))) && (((desired==CurrentRate) == (false)))]
  (junction 1073758490) -> (junction 1073758498) [order 2]
  (junction 1073758492) -> (junction 1073758494) : {
      | reqtable_postcondition((((adjust) == ("down"))), 'R:2.1');
      |
      |
      | }
  (junction 1073758494) -> (junction 1073758496) : {
      | }
  (junction 1073758496) -> (junction 1073758498)
  (junction 1073758498) -> (junction 1073758500)
  (junction 1073758500) -> (junction 1073758502) : {
      | % END_R_148
      | }
  (junction 1073758502) -> (junction 1073758504) : {
      | % START_R_151
      | }
  (junction 1073758504) -> (junction 1073758506) : {
      | }
  (junction 1073758506) -> (junction 1073758508)
  (junction 1073758508) -> (junction 1073758510) [order 1] : [(((desired<CurrentRate) == (false))) && (((desired>CurrentRate) == (true))) && (((desired==CurrentRate) == (false)))]
  (junction 1073758508) -> (junction 1073758516) [order 2]
  (junction 1073758510) -> (junction 1073758512) : {
      | reqtable_postcondition((((adjust) == ("up"))), 'R:2.2');
      |
      |
      | }
  (junction 1073758512) -> (junction 1073758514) : {
      | }
  (junction 1073758514) -> (junction 1073758516)
  (junction 1073758516) -> (junction 1073758518)
  (junction 1073758518) -> (junction 1073758520) : {
      | % END_R_151
      | }
  (junction 1073758520) -> (junction 1073758522) : {
      | % START_R_154
      | }
  (junction 1073758522) -> (junction 1073758524) : {
      | }
  (junction 1073758524) -> (junction 1073758526)
  (junction 1073758526) -> (junction 1073758528) [order 1] : [(((desired<CurrentRate) == (false))) && (((desired>CurrentRate) == (false))) && (((desired==CurrentRate) == (true)))]
  (junction 1073758526) -> (junction 1073758534) [order 2]
  (junction 1073758528) -> (junction 1073758530) : {
      | reqtable_postcondition((((adjust) == ("hold"))), 'R:2.3');
      |
      |
      | }
  (junction 1073758530) -> (junction 1073758532) : {
      | }
  (junction 1073758532) -> (junction 1073758534)
  (junction 1073758534) -> (junction 1073758536)
  (junction 1073758536) -> (junction 1073758538) : {
      | % END_R_154
      | }
  (junction 1073758538) -> (junction 1073758540)
  (junction 1073758540) -> (junction 1073758542)
  (junction 1073758542) -> (junction 1073758544) : {
      | % END_R_145
      | }
  (junction 1073758544) -> (junction 1073758546) : {
      | % START_R_157
      | }
  (junction 1073758546) -> (junction 1073758548) : {
      | }
  (junction 1073758548) -> (junction 1073758550)
  (junction 1073758550) -> (junction 1073758552) [order 1] : [(((mode) >= (0) && (mode) <= (8)))]
  (junction 1073758550) -> (junction 1073758558) [order 2]
  (junction 1073758552) -> (junction 1073758554) : {
      | reqtable_postcondition((((comparator) == ("below")) || ((comparator) == ("within")) || ((comparator) == ("above")) || ((comparator) == (""))) && (((adjust) == ("down")) || ((adjust) == ("up")) || ((adjust) == ("hold")) || ((adjust) == (""))), 'R:3');
      |
      |
      | }
  (junction 1073758554) -> (junction 1073758556) : {
      | }
  (junction 1073758556) -> (junction 1073758558)
  (junction 1073758558) -> (junction 1073758560)
  (junction 1073758560) -> (junction 1073758562) : {
      | % END_R_157
      | }
  data: LRL input double; URL input double; mode input int16; adjust input string; threshold input double; CurrentRate input double; RecoveryTime input double; level input double; desired input double; resp_factor input double; ReactionTime input double; comparator input string; MSR_level input double
